simulink model "SERIAL_TRANSMIT_VCPEPF"  (R2021b)
settings: Solver=FixedStepAuto  StartTime=0.0  StopTime=inf  RelTol=1e-3  EnableMultiTasking=on
model workspace (MAT data in the model file):
  x = 1
libraries: arduinolib x2, dspstat3 x2, simulink x1
settings Model: ExtModeTrigDuration=2  Creator=kisho  LastModifiedBy=kisho
settings OptimizationCC: EnhancedBackFolding=on  PassReuseOutputArgsAs=Individual arguments  ZeroExternalMemoryAtStartup=off  ZeroInternalMemoryAtStartup=off  MaxStackSize=64  OptimizeBlockOrder=speed  DifferentSizesBufferReuse=on  OptimizationCustomize=off  EfficientTunableParamExpr=on
settings DebuggingCC: ParameterTunabilityLossMsg=error
settings HardwareCC: ProdBitPerInt=16  ProdBitPerPointer=16  ProdBitPerSizeT=16  ProdBitPerPtrDiffT=16  ProdLargestAtomicFloat=None  ProdWordSize=8  ProdHWDeviceType=Atmel->AVR
settings SFSimCC: MATLABDynamicMemAlloc=off
settings RTWCC: Description=Embedded Coder  SystemTargetFile=ert.tlc  HardwareBoard=Arduino Mega 2560  TemplateMakefile=ert_default_tmf  Toolchain=Arduino AVR  BuildConfiguration=Faster Runs
settings CodeAppCC: ForceParamTrailComments=on  IgnoreCustomStorageClasses=off  OperatorAnnotations=on  SimulinkDataObjDesc=on  SFDataObjDesc=on  InsertBlockDesc=on
settings ERTTargetCC: SupportContinuousTime=on  SupportVariableSizeSignals=on  ExtModeTransport=3  ExtModeStaticAlloc=on  ExtModeStaticAllocSize=2048  ExtModeMexFile=ext_xcp  ExtModeIntrfLevel=Level2 - Open

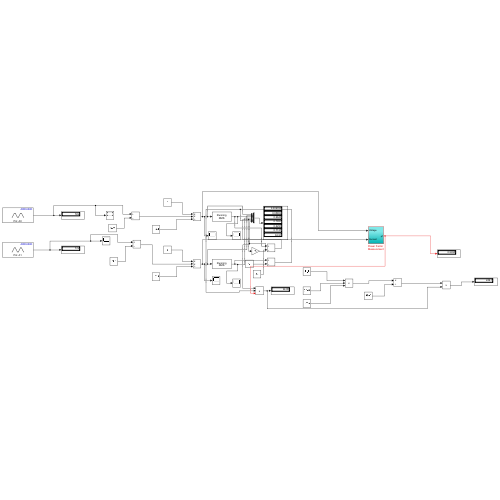
[thumbnail: Simulink's stored preview of the top-level diagram]
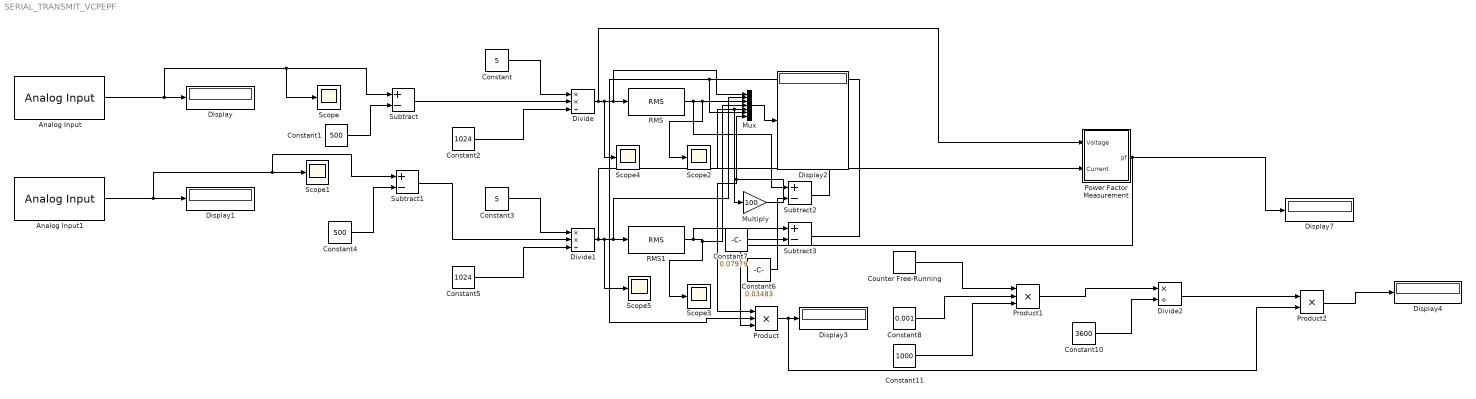
== system SERIAL_TRANSMIT_VCPEPF ==
  Analog Input : arduinolib/Analog Input  pinNumber=0  ReadResultsOnly=off  ConversionTriggerSource=Software  ExternalTriggerType=uint32( 0 )  OutputDataType=uint16  EnableConversionCompleteNotify=off  EnableOuputStatus=off  SampleTime=0.001  blockPlatform=arduino
  Analog Input1 : arduinolib/Analog Input  pinNumber=1  ReadResultsOnly=off  ConversionTriggerSource=Software  ExternalTriggerType=uint32( 0 )  OutputDataType=uint16  EnableConversionCompleteNotify=off  EnableOuputStatus=off  SampleTime=0.001  blockPlatform=arduino
  Constant : Constant  Value=5
  Constant1 : Constant  Value=500
  Constant10 : Constant  Value=3600
  Constant11 : Constant  Value=1000
  Constant2 : Constant  Value=1024
  Constant3 : Constant  Value=5
  Constant4 : Constant  Value=500
  Constant5 : Constant  Value=1024
  Constant6 : Constant  Value=0.03483
  Constant7 : Constant  Value=0.07979
  Constant8 : Constant  Value=0.001
  Counter Free-Running : simulink/Sources/Counter Free-Running  NumBits=32  tsamp=0.001
  Display{,1..4,7} (6 alike) : Display
  Divide : Product  Inputs=**/
  Divide1 : Product  Inputs=**/
  Divide2 : Product  Inputs=*/
  Multiply : Gain  Gain=100
  Mux : Mux  Inputs=7
  Power Factor Measurement : Subsystem
  Product : Product  Inputs=3  OutDataTypeStr=double
  Product1 : Product  Inputs=3
  Product2 : Product
  RMS : dspstat3/RMS  run=on  directionMode=Each column  dimension=1  InputProcessing=Columns as channels (frame based)  reset_popup=None
  RMS1 : dspstat3/RMS  run=on  directionMode=Each column  dimension=1  InputProcessing=Columns as channels (frame based)  reset_popup=None
  Scope{,1..5} (6 alike) : Scope
  Subtract{,1..3} (4 alike) : Sum  Inputs=+-
  wires:
  Constant/1 -> Divide/1
  Constant2/1 -> Divide/3
  RMS/1 -> Mux/3, Scope2/1, Subtract2/1
  Constant3/1 -> Divide1/1
  Analog Input1/1 -> Subtract1/1, Scope1/1, Display1/1
  Constant5/1 -> Divide1/3
  RMS1/1 -> Subtract3/1, Scope3/1, Mux/4
  Analog Input/1 -> Subtract/1, Scope/1, Display/1
  Mux/1 -> Display2/1
  Subtract/1 -> Divide/2
  Constant1/1 -> Subtract/2
  Subtract1/1 -> Divide1/2
  Constant4/1 -> Subtract1/2
  Subtract2/1 -> Multiply/1, Mux/5
  Constant6/1 -> Subtract2/2
  Constant7/1 -> Subtract3/2
  Counter Free-Running/1 -> Product1/1
  Divide2/1 -> Product2/1
  Constant8/1 -> Product1/2
  Constant10/1 -> Divide2/2
  Product1/1 -> Divide2/1
  Product/1 -> Product2/2, Display3/1
  Constant11/1 -> Product1/3
  Subtract3/1 -> Product/2, Mux/6
  Multiply/1 -> Mux/7, Product/1
  Divide/1 -> Power Factor Measurement/1(Voltage), Scope4/1, Mux/1, RMS/1
  Divide1/1 -> RMS1/1, Mux/2, Scope5/1, Power Factor Measurement/2(Current)
  Power Factor Measurement/1(pf) -> Display7/1, Product/3
  Product2/1 -> Display4/1

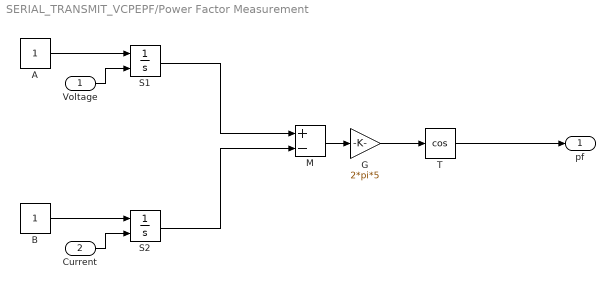
== system SERIAL_TRANSMIT_VCPEPF/Power Factor Measurement ==
  Voltage : Inport
  Current : Inport  Port=2
  A : Constant
  B : Constant
  G : Gain  Gain=2*pi*5
  M : Sum  Inputs=+-
  S1 : Integrator  ExternalReset=falling
  S2 : Integrator  ExternalReset=falling
  T : Trigonometry  Operator=cos
  pf : Outport
  wires:
  A/1 -> S1/1
  B/1 -> S2/1
  S1/1 -> M/1
  S2/1 -> M/2
  Voltage/1 -> S1/2
  Current/1 -> S2/2
  M/1 -> G/1
  G/1 -> T/1
  T/1 -> pf/1
